simulink model "New_com_Fixed_Angle"  (R2025a)
settings: Solver=VariableStepAuto  StartTime=0.0  StopTime=Inf  RelTol=1e-3
values from neighbouring files (symbols this model uses):
  Boom_Cmd_LUT = joints(1).lut_y    [LUT.m]
  Boom_Vel_LUT = joints(1).lut_x    [LUT.m]
  Stick_Cmd_LUT = joints(2).lut_y    [LUT.m]
  Stick_Vel_LUT = joints(2).lut_x    [LUT.m]
undefined symbols (not defined in the file or in its folder): canChannel
libraries: canlib x10, canmsglib x8, simulink_extras x6, simulink x6, eeGeneralControl x5, slpidlib x5, aerolibanimutils x1, sl3dlib x1
(part 1 of 2)
settings Model: Creator=Viktor Traktor  LastModifiedBy=Viktor Traktor

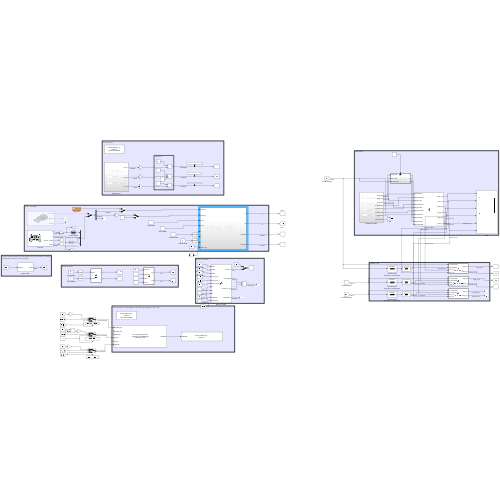
[thumbnail: Simulink's stored preview of the top-level diagram]
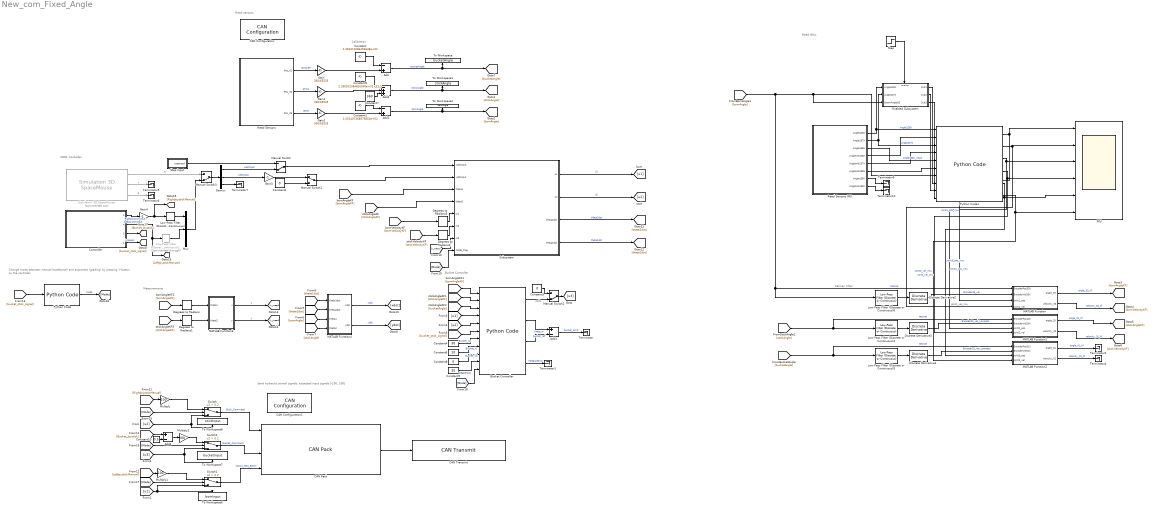
== system New_com_Fixed_Angle ==
  note: Change mode between manual (traditional) and automatic (grading)
      | by pressing Y-button on the controller
  note: Measurements
  note: Bucket Controller
  note: 2DOF Controller
  note: Calibration
  note: Send hydraulic control signals, expected input signals [-100, 100]
  note: Read sensors
  note: Kalman Filter
  note: Read IMUs
  Add : Sum  Inputs=-+
  Add1 : Sum  Inputs=+-
  Add2 : Sum  Inputs=-+
  Add3 : Sum  Inputs=-++
  Add4 : Sum  Inputs=+-
  Bucket Controller : PythonCode  OutputCode=|  SampleTime=0.01
      | import numpy as np
      | from numpy import sign, abs
      | 
      | #### TUNING PARAMETERS
      | degpersec 
      | Ts = 0.01
      | 
      | BUCKET_STICK1 = 16
      | BUCKET_STICK2 = 32
      | if flag is None:
      |     flag = 1
      | 
      | ## Bucket Control Parameters
      | Kp_bucket = Kp
      | Ki_bucket = Ki
      | Kd_bucket = Kd
      | 
      | ## Bucket controller
      | calc_thetaw = theta1 + theta2 + theta3
      | 
      | 
      | if theta_ref is None:
      |     theta_ref = -20
      | 
      | if comp_flag_1 is None:
      |     comp_flag_1 = 0
      | 
      |     
      | 
      | 
      | if bucket_stick_signal == 0 and flag == 0:
      |     if comp_flag_1 == 1:
      |         theta_ref = calc_thetaw - 0.6
      |     else:
      |         theta_ref = calc_thetaw + 0.6
      |     bucket_error_integral_prev = 0
      |     bucket_error_integral = 0
      |     bucket_error_prev = 0
      |     flag = 1
      |     
      | 
      | if bucket_stick_signal == BUCKET_STICK1 or bucket_stick_signal == BUCKET_STICK2:
      |     if bucket_stick_signal == BUCKET_STICK1 + BUCKET_STICK2:
      |         pass
      |     else:
      | 
      |         flag = 0
      | 
      |         if bucket_stick_signal == BUCKET_STICK1:
      |             theta_ref -= degpersec * Ts 
      |             comp_flag_1 = 1
      | 
      |         elif bucket_stick_signal == BUCKET_STICK2:
      |             theta_ref += degpersec * Ts 
      |             comp_flag_1 = 0
      |     
      | bucket_error = theta_ref - calc_thetaw
      | 
      | if bucket_error_prev is None:
      |     bucket_error_prev = bucket_error
      | if bucket_error_integral_prev is None:
      |     bucket_error_integral_prev  = 0
      | 
      | # calculate integral
      | if mode_flag == 1:
      |     
      |     bucket_error_integral = 0
      |     bucket_error_integral_prev = 0
      | 
      | else:
      |     bucket_error_integral = (bucket_error + bucket_error_prev) * Ts / 2 + bucket_error_integral_prev
      | 
      |     bucket_error_integral_prev = bucket_error_integral
      | 
      | 
      | # calculate derivative
      | bucket_error_derivative = (bucket_error - bucket_error_prev) / Ts
      | bucket_error_prev = bucket_error
      | 
      | 
      | control_3 = -(Kp_bucket * bucket_error +  Ki_bucket * bucket_error_integral +  Kd_bucket * bucket_error_derivative  + 0.2*stick_input + 0.2*bom_input)
      | control_3 = np.clip(control_3,-99, 90)
      | #if control_3 < 0:
      | #    control_3 = control_3 * 0.85 - 15
      | #else:
      | #    control_3 = control_3 * 0.85 + 15
      |             
      | bucket_ref_out = theta_ref
      | 
      | IntegralError = bucket_error_integral
  CAN Configuration : canlib/CAN Configuration  BlockHandle=316.0001  Device=Kvaser USBcan Light 1 (Channel 1)  DeviceMenu=Kvaser USBcan Light 1 (Channel 1)  ObjConstructor=canChannel('Kvaser', 'USBcan Light 1', 1)  BusSpeed=500000  EnableBitParameters=off  SJW=1  TSEG1=4  TSEG2=3  NSamples=1  AckMode=Normal
  CAN Configuration1 : canlib/CAN Configuration  BlockHandle=317.0001  Device=Kvaser USBcan Light 1 (Channel 2)  DeviceMenu=Kvaser USBcan Light 1 (Channel 2)  ObjConstructor=canChannel('Kvaser', 'USBcan Light 1', 2)  BusSpeed=500000  EnableBitParameters=off  SJW=1  TSEG1=4  TSEG2=3  NSamples=1  AckMode=Normal
  CAN Pack : canmsglib/CAN Pack  CANdbFile=C:\Users\Viktor Traktor\IQAN\ec20_hydraulics.dbc  MsgList=ControlMessage  MsgName=ControlMessage  MsgIDType=Standard (11-bit identifier)  MsgIdentifier=387  CANIDInput=off  MsgLength=6  Remote=off  ApplyMinMax=off  BusOutput=off  SignalInfo={'Parallell_FR','8','8','LE','signed','Standard','0','1','0','-Inf','Inf';'Parallelll_RL','0','8','LE','signed','Standard','0','1','0','-Inf','Inf';'Rotate_RL','40','8','LE','signed','Standard','0','1','0','-Inf','Inf';'Tilt_FR','24','8','LE','signed','Standard','0','1','0','-Inf','Inf';'Tilt_RL','32','8','LE','signed','Standard','0','1','0','-Inf','Inf';'UpDown','16','8','LE','signed','Standard','0','1','0','-Inf','Inf'}
      settings: LibrarySourceBlock=canlib/CAN Pack  DataFormat=CANdb specified signals
  CAN Transmit : canlib/CAN Transmit  BlockHandle=326.0001  Device=Kvaser USBcan Light 1 (Channel 2)  DeviceMenu=Kvaser USBcan Light 1 (Channel 2)  ObjConstructor=canChannel('Kvaser', 'USBcan Light 1', 2)  EnableEventTransmit=off  EnablePeriodicTransmit=off  MessagePeriod=1.000
  Constant : Constant  Value=2.060410383456638e+02
  Constant1 : Constant  Value=2.052407368979854e+02
  Constant10 : Constant  Value=0.5
  Constant2 : Constant  Value=0
  Constant3 : Constant  Value=0
  Constant4 : Constant  Value=30
  Constant5 : Constant  Value=2.390501084826040e+02+27.5
  Constant6 : Constant  Value=10
  Constant7 : Constant  Value=360
  Constant8 : Constant  Value=0
  Constant9 : Constant  Value=30
  Controller : Subsystem
      mask Display: image('controller.png', [0,0,20,0,100,100]);
  Degrees to Radians{,1..2,5} (4 alike) : simulink_extras/Transformations/Degrees to Radians
  Demux : Demux  Outputs=3
  Discrete Derivative2 : simulink/Discrete/Discrete Derivative  gainval=1.0  ICPrevScaledInput=0.0  OutMin=[]  OutMax=[]  OutDataType=fixdt(1, 16)  OutScaling=2^-10  DoSatur=off
  Discrete Derivative3 : simulink/Discrete/Discrete Derivative  gainval=1.0  ICPrevScaledInput=0.0  OutMin=[]  OutMax=[]  OutDataType=fixdt(1, 16)  OutScaling=2^-10  DoSatur=off
  Discrete Derivative4 : simulink/Discrete/Discrete Derivative  gainval=1.0  ICPrevScaledInput=0.0  OutMin=[]  OutMax=[]  OutDataType=fixdt(1, 16)  OutScaling=2^-10  DoSatur=off
  Enabled Subsystem : Subsystem  TreatAsAtomicUnit=on
  Gain : Gain  Gain=360/65535
  Gain1 : Gain  Gain=360/65535
  Gain2 : Gain  Gain=360/65535
  Gain3 : Gain  Gain=-1
  Gain4 : Gain  Gain=-1
  IMU : Scope  NumInputPorts=6
      settings: ActiveDisplayYMinimum=240.03476604985391  ActiveDisplayYMaximum=241.62685406904103
  Low-Pass Filter (Discrete or Continuous) : eeGeneralControl/Low-Pass Filter (Discrete or Continuous)  K=1  T=0.2  B=inf  A=-inf  init_option=Inherited from block input  x0=0  Ts=-1
  Low-Pass Filter (Discrete or Continuous)1 : eeGeneralControl/Low-Pass Filter (Discrete or Continuous)  Commented=through  K=1  T=0.2  B=inf  A=-inf  init_option=Inherited from block input  x0=0  Ts=-1
  Low-Pass Filter (Discrete or Continuous)4 : eeGeneralControl/Low-Pass Filter (Discrete or Continuous)  K=1  T=.15  B=inf  A=-inf  init_option=Inherited from block input  x0=0  Ts=0.1
  Low-Pass Filter (Discrete or Continuous)5 : eeGeneralControl/Low-Pass Filter (Discrete or Continuous)  K=1  T=.15  B=inf  A=-inf  init_option=Inherited from block input  x0=0  Ts=0.1
  Low-Pass Filter (Discrete or Continuous)6 : eeGeneralControl/Low-Pass Filter (Discrete or Continuous)  K=1  T=.15  B=inf  A=-inf  init_option=Inherited from block input  x0=0  Ts=0.1
  MATLAB Function : MATLAB Function  TreatAsAtomicUnit=on
  MATLAB Function1 : MATLAB Function  TreatAsAtomicUnit=on
  MATLAB Function2 : MATLAB Function  TreatAsAtomicUnit=on
  MATLAB Function3 : MATLAB Function  TreatAsAtomicUnit=on
  MATLAB Function4 : MATLAB Function  TreatAsAtomicUnit=on
  Manual Switch : ManualSwitch  CurrentSetting=0
  Manual Switch1 : ManualSwitch
  Manual Switch2 : ManualSwitch  CurrentSetting=0
  Manual Switch3 : ManualSwitch  CurrentSetting=0
  Multiply : Gain  Gain=100
  Multiply1 : Gain  Gain=100
  Multiply2 : Gain  Gain=200
  Mux : Mux  Inputs=3
  Python Code : PythonCode  OutputCode=|
      | if flag is None:
      |     flag = 1
      |     mode = 0
      | 
      | # Detect button press
      | if knapp_Y == 8 and flag == 1:
      |     mode = 1 if mode == 0 else 0  # toggle mode
      |     flag = 0                       # mark the press as handled
      | 
      | 
      | # Reset the flag when button is released
      | if knapp_Y != 8:
      |     flag = 1
  Python Code1 : PythonCode  OutputCode=|  SampleTime=0.01
      | # Computation
      | 
      | #print(Angle128X)
      | 
      | if Angle128X > 180:
      |     Angle128X = abs(Angle128X) - 360
      |     
      | if Angle137X < 20:
      |     Angle137X = abs(Angle137X)+360
      |     
      | if Angle138X > 270:
      |     Angle138X = abs(Angle138X) - 360
      |     
      | #print("///")
      | #print(Angle128X)
      | 
      | print(Angle128Xp)
      | print(Angle137Xp)
      | print(Encoder33Xp)
      |     
      | joint1_pos = Angle137X -270 + Angle128X - (Angle137Xp-270 + Angle128Xp - Encoder33Xp)
      | joint1_vel = -(AngleVel137X - AngleVel128X)
      | 
      | joint2_pos = 180 + (90 - joint1_pos) + Angle138X
      | joint2_vel = AngleVel138X - joint1_vel
      | 
      | joint3_pos = 0
      | joint3_vel = 0
  Read Sensors : Subsystem
  Read Sensors IMU : Subsystem
  Simulation 3D SpaceMouse : sl3dlib/Simulation 3D/Hardware Interface/Simulation 3D SpaceMouse  Commented=on  Port=USB1  OutputType=Speed  Dominant=off  DisableTranslation=off  DisableRotation=off  NormalizeAngle=off  EnableLimit=off  PositionSensitivity=0.00058  RotationSensitivity=0.00001  InitialPosition=[0 0 0]  InitialRotation=[0 0 1 0]  PositionLow=[-100 -100 -100]  PositionUp=[100 100 100]
  Step : Step  Time=0.001  Before=1  After=0  SampleTime=0
  Step Input : Subsystem
  Subsystem : Subsystem
  Switch : Switch  Criteria=u2 > Threshold  Threshold=0.2  SaturateOnIntegerOverflow=off  InputSameDT=off
  Switch1 : Switch  Criteria=u2 > Threshold  Threshold=0.2  SaturateOnIntegerOverflow=off  InputSameDT=off
  Switch2 : Switch  Criteria=u2 > Threshold  Threshold=0.2  SaturateOnIntegerOverflow=off  InputSameDT=off
  Terminator{,1..2,4..7,9..10} (9 alike) : Terminator
  To Workspace : ToWorkspace  VariableName=bucketAngle  SaveFormat=Timeseries  SampleTime=-1
  To Workspace1 : ToWorkspace  VariableName=stickAngle  SaveFormat=Timeseries  SampleTime=-1
  To Workspace2 : ToWorkspace  VariableName=bomAngle  SaveFormat=Timeseries  SampleTime=-1
  To Workspace6 : ToWorkspace  VariableName=bomInput  SaveFormat=Timeseries  SampleTime=-1
  To Workspace7 : ToWorkspace  VariableName=bucketInput  SaveFormat=Timeseries  SampleTime=-1
  To Workspace8 : ToWorkspace  VariableName=stickInput  SaveFormat=Timeseries  SampleTime=-1
  wires:
  [u3] -> Switch2/3, To Workspace7/1
  Add2/1 -> [bomAngle], To Workspace2/1  "bomAngle"
  Constant1/1 -> Add2/1
  Gain/1 -> Add/2
  Read Sensors/2(Pos_20) -> Gain1/1  "STICK"
  [u2] -> To Workspace8/1, Switch/3
  Constant/1 -> Add/1
  Read Sensors/1(Pos_01) -> Gain/1  "BUCKET"
  Gain2/1 -> Add2/2
  Read Sensors/3(Pos_33) -> Gain2/1  "BOM"
  CAN Pack/1 -> CAN Transmit/1
  Add/1 -> [bucketAngle], To Workspace/1  "bucketAngle"
  [u1] -> To Workspace6/1, Switch1/3
  Add3/1 -> [stickAngle], To Workspace1/1  "stickAngle"
  MATLAB Function1/2(velocity_20) -> [stickVelocityKF]  "velocity_20_kf"
  Enabled Subsystem/1(Out1) -> Python Code1/8
  Discrete Derivative2/1 -> MATLAB Function/2(EncoderVel33X)  "Encoder33_vel"
  MATLAB Function/1(angle_33) -> [bomAngleKF]  "angle_33_kf"
  Read Sensors IMU/3(Angle138X) -> Python Code1/5  "Angle138X_input"
  Python Code1/4 -> MATLAB Function1/4(joint2_vel), IMU/4  "join2_vel_imu"
  Read Sensors IMU/4(AngleVel128X) -> Python Code1/2
  Read Sensors IMU/1(Angle128X) -> Python Code1/1, Enabled Subsystem/1(Angle128X)  "Angle128X"
  Read Sensors IMU/8(AngleVel139X) -> Terminator10/1
  Python Code1/3 -> MATLAB Function1/3(joint2_pos), IMU/3  "joint2_pos_imu"
  Python Code1/5 -> MATLAB Function2/3(joint3_pos), IMU/5  "joint3_pos_imu"
  MATLAB Function/2(velocity_33) -> [bomVelocityKF]  "velocity_33_kf"
  Python Code1/6 -> MATLAB Function2/4(joint3_vel), IMU/6  "joint3_vel_imu"
  Python Code1/2 -> MATLAB Function/4(joint1_vel), IMU/2  "joint1_vel_imu"
  MATLAB Function1/1(angle_20) -> [stickAngleKF]  "anlge_20_kf"
  Enabled Subsystem/3(Out3) -> Python Code1/10
  Read Sensors IMU/2(Angle137X) -> Python Code1/3, Enabled Subsystem/2(Angle137X)  "Angle137X"
  Step/1 -> Enabled Subsystem/Enable
  Discrete Derivative3/1 -> MATLAB Function1/2(EncoderVel20X)  "Encoder20_vel_Lowpass"
  Read Sensors IMU/5(AngleVel137X) -> Python Code1/4
  Python Code1/1 -> MATLAB Function/3(joint1_pos), IMU/1  "joint1_pos_imu"
  MATLAB Function2/1(angle_01) -> Terminator2/1  "angle_01_kf"
  Read Sensors IMU/7(Angle139X) -> Terminator9/1
  MATLAB Function2/2(velocity_01) -> Terminator4/1  "velocity_01_kf"
  Read Sensors IMU/6(AngleVel138X) -> Python Code1/6
  Enabled Subsystem/2(Out2) -> Python Code1/9
  Discrete Derivative4/1 -> MATLAB Function2/2(EncoderVel01X)  "Encoder01_vel_Lowpass"
  Constant5/1 -> Add3/1
  Gain1/1 -> Add3/2
  Constant7/1 -> Add3/3
  [stickAngle] -> MATLAB Function1/1(EncoderPos20X), Low-Pass Filter (Discrete or Continuous)4/1  "testvel"
  [bomAngle] -> Low-Pass Filter (Discrete or Continuous)6/1, MATLAB Function/1(EncoderPos33X), Python Code1/7, Enabled Subsystem/3(BoomAngle33)  "testvel"
  [bucketAngle] -> MATLAB Function2/1(EncoderPos01X), Low-Pass Filter (Discrete or Continuous)5/1  "testvel"
  Low-Pass Filter (Discrete or Continuous)5/1 -> Discrete Derivative4/1
  Low-Pass Filter (Discrete or Continuous)4/1 -> Discrete Derivative3/1
  Low-Pass Filter (Discrete or Continuous)6/1 -> Discrete Derivative2/1
  Simulation 3D SpaceMouse/1 -> Manual Switch3/1  "tr"
  Subsystem/2(u2) -> [u2]  "u2"
  Demux/2 -> Gain3/1  "ydotInput"
  Demux/1 -> Manual Switch/2  "xdotInput"
  Simulation 3D SpaceMouse/2 -> Terminator5/1  "r"
  Simulation 3D SpaceMouse/3 -> Terminator6/1  "b"
  Subsystem/1(u1) -> [u1]  "u1"
  Gain3/1 -> Manual Switch1/1
  [bomAngleKF] -> Subsystem/3(theta1)
  [stickAngleKF] -> Subsystem/4(theta2)
  Degrees to Radians2/1 -> Subsystem/6(In2)
  [stickVelocityKF] -> Degrees to Radians2/1
  [bomVelocityKF] -> Degrees to Radians5/1
  Degrees to Radians5/1 -> Subsystem/5(In1)
  Step Input/1(stepInput) -> Manual Switch/1
  Manual Switch/1 -> Subsystem/1(xdotInput)
  Constant2/1 -> Manual Switch1/2
  Manual Switch1/1 -> Subsystem/2(ydotInput)
  Controller/2(4) -> Low-Pass Filter (Discrete or Continuous)1/1, [LeftJoystickManual]  "LeftJoystckInput"
  Controller/1(2) -> Gain4/1  "RightJoystickInput"
  Gain4/1 -> [RightJoystickManual], Low-Pass Filter (Discrete or Continuous)/1
  Mux/1 -> Manual Switch3/2
  Manual Switch3/1 -> Demux/1
  Controller/4(1) -> [bucket_stick_signal]  "knappar"
  Demux/3 -> Terminator7/1
  Subsystem/3(theta2dot) -> [theta2dot]  "theta2dot"
  Subsystem/4(theta1dot) -> [theta1dot]  "theta1dot"
  [y_meas] -> Subsystem/7(In3)
  Constant3/1 -> Manual Switch2/1
  [stickAngleKF] -> Bucket Controller/2
  [bomAngleKF] -> Bucket Controller/1
  [bucketAngle] -> Bucket Controller/3
  [u2] -> Bucket Controller/5
  [u1] -> Bucket Controller/4
  Bucket Controller/2 -> Add1/1  "theta_w"
  Manual Switch2/1 -> [u3]
  [bucket_stick_signal] -> Bucket Controller/6
  Bucket Controller/1 -> Manual Switch2/2  "ctrl3"
  Degrees to Radians1/1 -> MATLAB Function3/2(theta2)
  [bomAngleKF] -> Degrees to Radians/1
  [bomAngle] -> MATLAB Function4/3(theta1)
  [theta2dot] -> MATLAB Function4/2(theta2dot)
  [stickAngleKF] -> Degrees to Radians1/1
  MATLAB Function3/1(x) -> [x_meas]  "x"
  MATLAB Function4/2(ydot) -> [ydot]  "ydot"
  [theta1dot] -> MATLAB Function4/1(theta1dot)
  MATLAB Function3/2(y) -> [y_meas]  "y"
  [stickAngle] -> MATLAB Function4/4(theta2)
  MATLAB Function4/1(xdot) -> [xdot]  "xdot"
  Degrees to Radians/1 -> MATLAB Function3/1(theta1)
  Constant4/1 -> Bucket Controller/7  "Bucket_kp"
  Constant6/1 -> Bucket Controller/8  "Bucket_ki"
  Constant8/1 -> Bucket Controller/9  "Bucket_kd"
  Bucket Controller/3 -> Add1/2  "bucket_ref"
  Constant9/1 -> Bucket Controller/10  "Degpersec"
  Low-Pass Filter (Discrete or Continuous)1/1 -> Mux/2
  Low-Pass Filter (Discrete or Continuous)/1 -> Mux/1
  Add1/1 -> Terminator/1  "bucket_error"
  Switch/1 -> CAN Pack/1  "Stick_Command"
  Multiply/1 -> Switch/1
  [LeftJoystickManual] -> Multiply1/1
  Switch1/1 -> CAN Pack/6  "Marko_test_Boom"
  Multiply1/1 -> Switch1/1
  [bucket_stick_signal] -> Python Code/1
  [RightJoystickManual] -> Multiply/1
  Controller/3(3) -> [Bucket_Joystick]
  Python Code/1 -> [Mode]  "Mode"
  [Mode] -> Switch/2
  Multiply2/1 -> Switch2/1
  [Mode] -> Switch2/2
  [Mode] -> Switch1/2
  Switch2/1 -> CAN Pack/4  "Bucket_Command"
  Add4/1 -> Multiply2/1
  [Bucket_Joystick] -> Add4/1
  Constant10/1 -> Add4/2
  [Mode] -> Bucket Controller/11
  Bucket Controller/4 -> Terminator1/1  "IntegralError"
  [Mode] -> Subsystem/8(Mode_Flag)

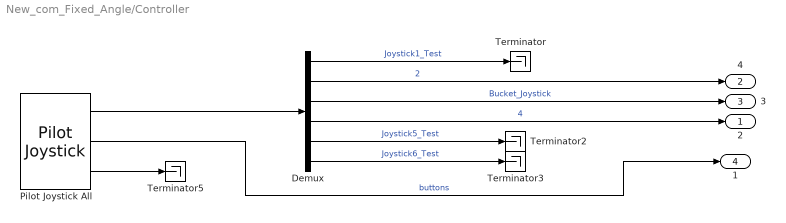
== system New_com_Fixed_Angle/Controller ==
  Demux : Demux  Outputs=6
  Pilot Joystick All : aerolibanimutils/Pilot Joystick  JoystickID=Joystick2  OutputConfiguration=AllOutputs  SampleTime=1/50
      settings: LibrarySourceBlock=aerolibanimutils/Pilot Joystick All
  Terminator{,2..3,5} (4 alike) : Terminator
  2 : Outport
  4 : Outport  Port=2
  3 : Outport  Port=3
  1 : Outport  Port=4
  wires:
  Demux/6 -> Terminator3/1  "Joystick6_Test"
  Demux/5 -> Terminator2/1  "Joystick5_Test"
  Pilot Joystick All/3 -> Terminator5/1
  Pilot Joystick All/1 -> Demux/1
  Demux/1 -> Terminator/1  "Joystick1_Test"
  Demux/4 -> 2/1  "4"
  Pilot Joystick All/2 -> 1/1  "buttons"
  Demux/3 -> 3/1  "Bucket_Joystick"
  Demux/2 -> 4/1  "2"

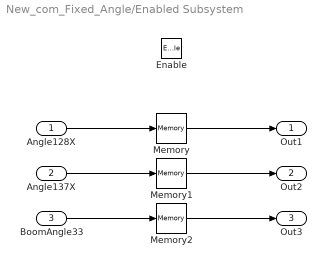
== system New_com_Fixed_Angle/Enabled Subsystem ==
  Angle128X : Inport
  Angle137X : Inport  Port=2
  BoomAngle33 : Inport  Port=3
  Enable : EnablePort
  Memory : Memory
  Memory1 : Memory
  Memory2 : Memory
  Out1 : Outport
  Out2 : Outport  Port=2
  Out3 : Outport  Port=3
  wires:
  Angle128X/1 -> Memory/1
  Memory/1 -> Out1/1
  Angle137X/1 -> Memory1/1
  BoomAngle33/1 -> Memory2/1
  Memory1/1 -> Out2/1
  Memory2/1 -> Out3/1

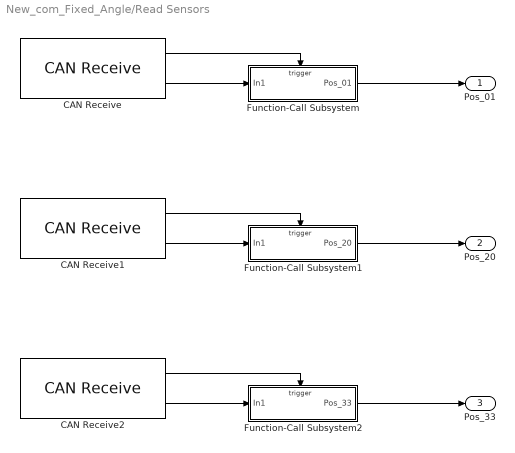
== system New_com_Fixed_Angle/Read Sensors ==
  CAN Receive : canlib/CAN Receive  BlockHandle=820.0001  Device=Kvaser USBcan Light 1 (Channel 1)  DeviceMenu=Kvaser USBcan Light 1 (Channel 1)  ObjConstructor=canChannel('Kvaser', 'USBcan Light 1', 1)  EnableStandardIDsFilter=off  StdIDsCombo=Allow all  StandardIDs=0  EnableExtendedIDsFilter=off  ExtIDsCombo=Allow all  ExtendedIDs=0  SampleTime=0.01  MsgsPerTimestep=all  InternalFilterUpdateStatus=on  BusOutput=off
  CAN Receive1 : canlib/CAN Receive  BlockHandle=823.0001  Device=Kvaser USBcan Light 1 (Channel 1)  DeviceMenu=Kvaser USBcan Light 1 (Channel 1)  ObjConstructor=canChannel('Kvaser', 'USBcan Light 1', 1)  EnableStandardIDsFilter=off  StdIDsCombo=Allow all  StandardIDs=0  EnableExtendedIDsFilter=off  ExtIDsCombo=Allow all  ExtendedIDs=0  SampleTime=0.01  MsgsPerTimestep=all  InternalFilterUpdateStatus=on  BusOutput=off
  CAN Receive2 : canlib/CAN Receive  BlockHandle=826.0001  Device=Kvaser USBcan Light 1 (Channel 1)  DeviceMenu=Kvaser USBcan Light 1 (Channel 1)  ObjConstructor=canChannel('Kvaser', 'USBcan Light 1', 1)  EnableStandardIDsFilter=off  StdIDsCombo=Allow all  StandardIDs=0  EnableExtendedIDsFilter=off  ExtIDsCombo=Allow all  ExtendedIDs=0  SampleTime=0.01  MsgsPerTimestep=all  InternalFilterUpdateStatus=on  BusOutput=off
  Function-Call Subsystem : Subsystem  TreatAsAtomicUnit=on
  Function-Call Subsystem1 : Subsystem  TreatAsAtomicUnit=on
  Function-Call Subsystem2 : Subsystem  TreatAsAtomicUnit=on
  Pos_01 : Outport
  Pos_20 : Outport  Port=2
  Pos_33 : Outport  Port=3
  wires:
  CAN Receive/2 -> Function-Call Subsystem/1(In1)
  CAN Receive1/2 -> Function-Call Subsystem1/1(In1)
  CAN Receive/1 -> Function-Call Subsystem/Trigger
  CAN Receive2/2 -> Function-Call Subsystem2/1(In1)
  Function-Call Subsystem2/1(Pos_33) -> Pos_33/1
  Function-Call Subsystem/1(Pos_01) -> Pos_01/1
  CAN Receive2/1 -> Function-Call Subsystem2/Trigger
  CAN Receive1/1 -> Function-Call Subsystem1/Trigger
  Function-Call Subsystem1/1(Pos_20) -> Pos_20/1

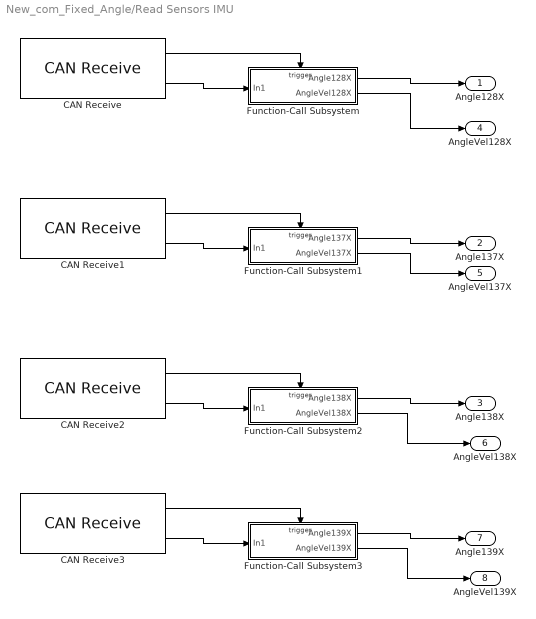
== system New_com_Fixed_Angle/Read Sensors IMU ==
  CAN Receive : canlib/CAN Receive  BlockHandle=907.0001  Device=Kvaser USBcan Light 1 (Channel 1)  DeviceMenu=Kvaser USBcan Light 1 (Channel 1)  ObjConstructor=canChannel('Kvaser', 'USBcan Light 1', 1)  EnableStandardIDsFilter=off  StdIDsCombo=Allow all  StandardIDs=0  EnableExtendedIDsFilter=off  ExtIDsCombo=Allow all  ExtendedIDs=0  SampleTime=0.01  MsgsPerTimestep=all  InternalFilterUpdateStatus=on  BusOutput=off
  CAN Receive1 : canlib/CAN Receive  BlockHandle=910.0001  Device=Kvaser USBcan Light 1 (Channel 1)  DeviceMenu=Kvaser USBcan Light 1 (Channel 1)  ObjConstructor=canChannel('Kvaser', 'USBcan Light 1', 1)  EnableStandardIDsFilter=off  StdIDsCombo=Allow all  StandardIDs=0  EnableExtendedIDsFilter=off  ExtIDsCombo=Allow all  ExtendedIDs=0  SampleTime=0.01  MsgsPerTimestep=all  InternalFilterUpdateStatus=on  BusOutput=off
  CAN Receive2 : canlib/CAN Receive  BlockHandle=913.0001  Device=Kvaser USBcan Light 1 (Channel 1)  DeviceMenu=Kvaser USBcan Light 1 (Channel 1)  ObjConstructor=canChannel('Kvaser', 'USBcan Light 1', 1)  EnableStandardIDsFilter=off  StdIDsCombo=Allow all  StandardIDs=0  EnableExtendedIDsFilter=off  ExtIDsCombo=Allow all  ExtendedIDs=0  SampleTime=0.01  MsgsPerTimestep=all  InternalFilterUpdateStatus=on  BusOutput=off
  CAN Receive3 : canlib/CAN Receive  BlockHandle=916.0001  Device=Kvaser USBcan Light 1 (Channel 1)  DeviceMenu=Kvaser USBcan Light 1 (Channel 1)  ObjConstructor=canChannel('Kvaser', 'USBcan Light 1', 1)  EnableStandardIDsFilter=off  StdIDsCombo=Allow all  StandardIDs=0  EnableExtendedIDsFilter=off  ExtIDsCombo=Allow all  ExtendedIDs=0  SampleTime=0.01  MsgsPerTimestep=all  InternalFilterUpdateStatus=on  BusOutput=off
  Function-Call Subsystem : Subsystem  TreatAsAtomicUnit=on
  Function-Call Subsystem1 : Subsystem  TreatAsAtomicUnit=on
  Function-Call Subsystem2 : Subsystem  TreatAsAtomicUnit=on
  Function-Call Subsystem3 : Subsystem  TreatAsAtomicUnit=on
  Angle128X : Outport
  Angle137X : Outport  Port=2
  Angle138X : Outport  Port=3
  AngleVel128X : Outport  Port=4
  AngleVel137X : Outport  Port=5
  AngleVel138X : Outport  Port=6
  Angle139X : Outport  Port=7
  AngleVel139X : Outport  Port=8
  wires:
  Function-Call Subsystem1/1(Angle137X) -> Angle137X/1
  CAN Receive1/1 -> Function-Call Subsystem1/Trigger
  CAN Receive2/1 -> Function-Call Subsystem2/Trigger
  Function-Call Subsystem/1(Angle128X) -> Angle128X/1
  Function-Call Subsystem2/1(Angle138X) -> Angle138X/1
  CAN Receive2/2 -> Function-Call Subsystem2/1(In1)
  CAN Receive/1 -> Function-Call Subsystem/Trigger
  CAN Receive1/2 -> Function-Call Subsystem1/1(In1)
  CAN Receive/2 -> Function-Call Subsystem/1(In1)
  Function-Call Subsystem/2(AngleVel128X) -> AngleVel128X/1
  Function-Call Subsystem1/2(AngleVel137X) -> AngleVel137X/1
  Function-Call Subsystem2/2(AngleVel138X) -> AngleVel138X/1
  Function-Call Subsystem3/2(AngleVel139X) -> AngleVel139X/1
  CAN Receive3/2 -> Function-Call Subsystem3/1(In1)
  Function-Call Subsystem3/1(Angle139X) -> Angle139X/1
  CAN Receive3/1 -> Function-Call Subsystem3/Trigger

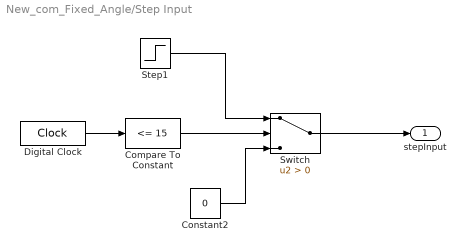
== system New_com_Fixed_Angle/Step Input ==
  Compare To Constant : simulink/Logic and Bit Operations/Compare To Constant  relop=<=  const=15  OutDataTypeStr=boolean
  Constant2 : Constant  Value=0
  Digital Clock : DigitalClock  SampleTime=0.01
  Step1 : Step  SampleTime=0.01
  Switch : Switch  Criteria=u2 > Threshold  SaturateOnIntegerOverflow=off  InputSameDT=off
  stepInput : Outport
  wires:
  Switch/1 -> stepInput/1
  Compare To Constant/1 -> Switch/2
  Digital Clock/1 -> Compare To Constant/1
  Step1/1 -> Switch/1
  Constant2/1 -> Switch/3

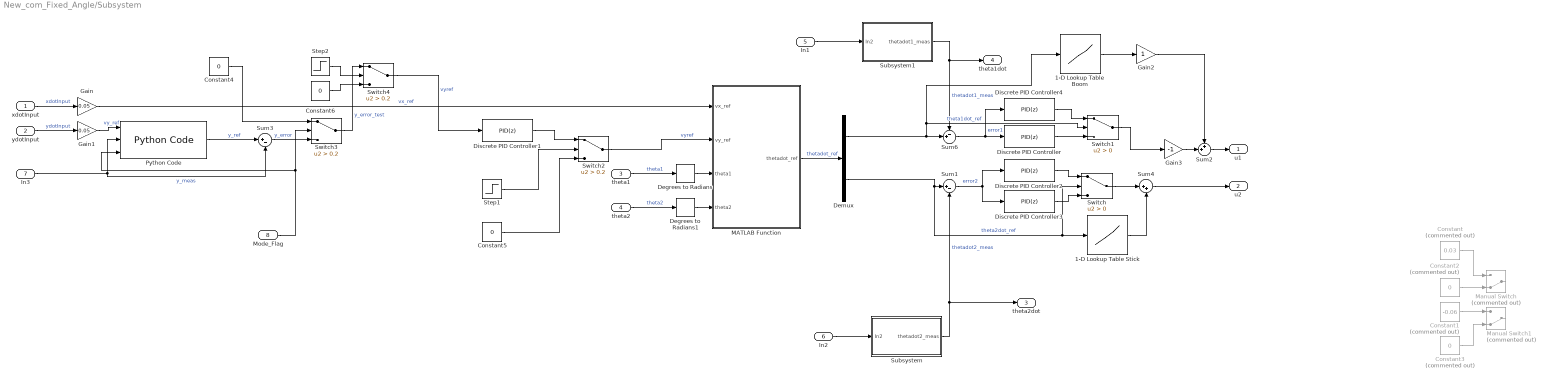
== system New_com_Fixed_Angle/Subsystem ==
  xdotInput : Inport
  ydotInput : Inport  Port=2
  theta1 : Inport  Port=3
  theta2 : Inport  Port=4
  In1 : Inport  Port=5
  In2 : Inport  Port=6
  In3 : Inport  Port=7
  Mode_Flag : Inport  Port=8
  1-D Lookup Table Boom : Lookup_n-D  NumberOfTableDimensions=1  BreakpointsForDimension1=Boom_Vel_LUT  Table=Boom_Cmd_LUT  InternalRulePriority=Speed  RndMeth=Simplest
  1-D Lookup Table Stick : Lookup_n-D  NumberOfTableDimensions=1  BreakpointsForDimension1=Stick_Vel_LUT  Table=Stick_Cmd_LUT  InternalRulePriority=Speed  RndMeth=Simplest
  Constant : Constant  Commented=on  Value=0.03
  Constant1 : Constant  Commented=on  Value=-0.06
  Constant2 : Constant  Commented=on  Value=0
  Constant3 : Constant  Commented=on  Value=0
  Constant4 : Constant  Value=0
  Constant5 : Constant  Value=0
  Constant6 : Constant  Value=0
  Degrees to Radians : simulink_extras/Transformations/Degrees to Radians
  Degrees to Radians1 : simulink_extras/Transformations/Degrees to Radians
  Demux : Demux  Outputs=2
  Discrete PID Controller : slpidlib/PID Controller  Controller=PID  Form=Parallel  TimeDomain=Discrete-time  UseExternalTs=off  SampleTime=-1  IntegratorMethod=Forward Euler  FilterMethod=Forward Euler  ControllerParametersSource=internal  P=75  I=100  UseKiTs=off  D=3  UseExternalDerivativeSource=off  N=100  UseFilter=on  TunerSelectOption=Transfer Function Based (PID Tuner App)  InitialConditionSource=internal  InitialConditionForIntegrator=0  InitialConditionForFilter=0  DifferentiatorICPrevScaledInput=0  ExternalReset=none  TrackingMode=off  Kt=1  LimitOutput=on  SatLimitsSource=internal  UpperSaturationLimit=100  LowerSaturationLimit=-100  LinearizeAsGain=off  AntiWindupMode=clamping  Kb=1  LimitIntegrator=on  UpperIntegratorSaturationLimit=50  LowerIntegratorSaturationLimit=-50  POutMin=[]  POutMax=[]  IOutMin=[]  IOutMax=[]  DOutMin=[]  DOutMax=[]  NOutMin=[]  NOutMax=[]  SumOutMin=[]  SumOutMax=[]  SaturationOutMin=[]  SaturationOutMax=[]  PParamMin=[]  PParamMax=[]  IParamMin=[]  IParamMax=[]  DParamMin=[]  DParamMax=[]  NParamMin=[]  NParamMax=[]  KbParamMin=[]  KbParamMax=[]  KtParamMin=[]  KtParamMax=[]  KbOutMin=[]  KbOutMax=[]  KtOutMin=[]  KtOutMax=[]  IntegratorOutMin=[]  IntegratorOutMax=[]  FilterOutMin=[]  FilterOutMax=[]  SumI1OutMin=[]  SumI1OutMax=[]  SumI2OutMin=[]  SumI2OutMax=[]  SumI3OutMin=[]  SumI3OutMax=[]  SumI4OutMin=[]  SumI4OutMax=[]  SumDOutMin=[]  SumDOutMax=[]  DifferentiatorOutMin=[]  DifferentiatorOutMax=[]  FilterDiffOutCoefMin=[]  FilterDiffOutCoefMax=[]  ReciprocalOutMin=[]  ReciprocalOutMax=[]  SumDenOutMin=[]  SumDenOutMax=[]  SumNumOutMin=[]  SumNumOutMax=[]  DivideOutMin=[]  DivideOutMax=[]  UdiffTsProdOutMin=[]  UdiffTsProdOutMax=[]  NTsProdOutMin=[]  NTsProdOutMax=[]  UintegralTsProdOutMin=[]  UintegralTsProdOutMax=[]  UngainTsProdOutMin=[]  UngainTsProdOutMax=[]  ClampingZeroOutDataTypeStr=Inherit: Inherit via back propagation  ClampingZeroOutMin=[]  ClampingZeroOutMax=[]  FilterDenConstantOutDataTypeStr=Inherit: Inherit via back propagation  FilterDenConstantOutMin=[]  FilterDenConstantOutMax=[]  PCopyOutDataTypeStr=Inherit: Inherit via back propagation  PCopyOutMin=[]  PCopyOutMax=[]  NCopyOutDataTypeStr=Inherit: Inherit via back propagation  NCopyOutMin=[]  NCopyOutMax=[]  IntegratorContinuousStateAttributes=''  IntegratorStateMustResolveToSignalObject=off  IntegratorRTWStateStorageClass=Auto  FilterContinuousStateAttributes=''  FilterStateMustResolveToSignalObject=off  FilterRTWStateStorageClass=Auto  ParallelPVariant=InternalParameters  IdealPVariant=Disabled  IVariant=InternalParameters  DVariant=InternalParameters  IntegratorVariant=Discrete  SatVariant=Enabled  AWVariant=DiscClampingParallel  PCopyVariant=Disabled  TRVariant=Disabled  FdbkBlocksVariant=Forward  IdealPFdbkVariant=Disabled  SatFdbkVariant=Disabled  DerivativeFilterVariant=ForwardEulerFilter  NVariant=InternalParameters  NCopyVariant=Disabled  FilterICVariant=InternalICsFilter  IntegratorICVariant=InternalICs  ExternalResetVariant=Disabled  TRSumVariant=Passthrough  SumFdbkVariant=Disabled  SumVariant=Sum_PID  TsampFilterVariant=InternalTs  TsampNgainVariant=Passthrough  TsampIntegralVariant=Disabled_SignalSpec  ExternalSaturationOutDataTypeStr=Inherit: Same as second input  DerivativeSourceVariant=ErrorSignal  PreIntVariant=InternalPreInt
      settings: LibrarySourceBlock=simulink/Discrete/Discrete PID Controller
  Discrete PID Controller1 : slpidlib/PID Controller  Controller=PID  Form=Parallel  TimeDomain=Discrete-time  UseExternalTs=off  SampleTime=-1  IntegratorMethod=Forward Euler  FilterMethod=Forward Euler  ControllerParametersSource=internal  P=1.3  I=0.8  UseKiTs=off  D=0  UseExternalDerivativeSource=off  N=30  UseFilter=on  TunerSelectOption=Transfer Function Based (PID Tuner App)  InitialConditionSource=internal  InitialConditionForIntegrator=0  InitialConditionForFilter=0  DifferentiatorICPrevScaledInput=0  ExternalReset=none  TrackingMode=off  Kt=1  LimitOutput=on  SatLimitsSource=internal  UpperSaturationLimit=100  LowerSaturationLimit=-100  LinearizeAsGain=off  AntiWindupMode=clamping  Kb=1  LimitIntegrator=on  UpperIntegratorSaturationLimit=50  LowerIntegratorSaturationLimit=-50  POutMin=[]  POutMax=[]  IOutMin=[]  IOutMax=[]  DOutMin=[]  DOutMax=[]  NOutMin=[]  NOutMax=[]  SumOutMin=[]  SumOutMax=[]  SaturationOutMin=[]  SaturationOutMax=[]  PParamMin=[]  PParamMax=[]  IParamMin=[]  IParamMax=[]  DParamMin=[]  DParamMax=[]  NParamMin=[]  NParamMax=[]  KbParamMin=[]  KbParamMax=[]  KtParamMin=[]  KtParamMax=[]  KbOutMin=[]  KbOutMax=[]  KtOutMin=[]  KtOutMax=[]  IntegratorOutMin=[]  IntegratorOutMax=[]  FilterOutMin=[]  FilterOutMax=[]  SumI1OutMin=[]  SumI1OutMax=[]  SumI2OutMin=[]  SumI2OutMax=[]  SumI3OutMin=[]  SumI3OutMax=[]  SumI4OutMin=[]  SumI4OutMax=[]  SumDOutMin=[]  SumDOutMax=[]  DifferentiatorOutMin=[]  DifferentiatorOutMax=[]  FilterDiffOutCoefMin=[]  FilterDiffOutCoefMax=[]  ReciprocalOutMin=[]  ReciprocalOutMax=[]  SumDenOutMin=[]  SumDenOutMax=[]  SumNumOutMin=[]  SumNumOutMax=[]  DivideOutMin=[]  DivideOutMax=[]  UdiffTsProdOutMin=[]  UdiffTsProdOutMax=[]  NTsProdOutMin=[]  NTsProdOutMax=[]  UintegralTsProdOutMin=[]  UintegralTsProdOutMax=[]  UngainTsProdOutMin=[]  UngainTsProdOutMax=[]  ClampingZeroOutDataTypeStr=Inherit: Inherit via back propagation  ClampingZeroOutMin=[]  ClampingZeroOutMax=[]  FilterDenConstantOutDataTypeStr=Inherit: Inherit via back propagation  FilterDenConstantOutMin=[]  FilterDenConstantOutMax=[]  PCopyOutDataTypeStr=Inherit: Inherit via back propagation  PCopyOutMin=[]  PCopyOutMax=[]  NCopyOutDataTypeStr=Inherit: Inherit via back propagation  NCopyOutMin=[]  NCopyOutMax=[]  IntegratorContinuousStateAttributes=''  IntegratorStateMustResolveToSignalObject=off  IntegratorRTWStateStorageClass=Auto  FilterContinuousStateAttributes=''  FilterStateMustResolveToSignalObject=off  FilterRTWStateStorageClass=Auto  ParallelPVariant=InternalParameters  IdealPVariant=Disabled  IVariant=InternalParameters  DVariant=InternalParameters  IntegratorVariant=Discrete  SatVariant=Enabled  AWVariant=DiscClampingParallel  PCopyVariant=Disabled  TRVariant=Disabled  FdbkBlocksVariant=Forward  IdealPFdbkVariant=Disabled  SatFdbkVariant=Disabled  DerivativeFilterVariant=ForwardEulerFilter  NVariant=InternalParameters  NCopyVariant=Disabled  FilterICVariant=InternalICsFilter  IntegratorICVariant=InternalICs  ExternalResetVariant=Disabled  TRSumVariant=Passthrough  SumFdbkVariant=Disabled  SumVariant=Sum_PID  TsampFilterVariant=InternalTs  TsampNgainVariant=Passthrough  TsampIntegralVariant=Disabled_SignalSpec  ExternalSaturationOutDataTypeStr=Inherit: Same as second input  DerivativeSourceVariant=ErrorSignal  PreIntVariant=InternalPreInt
      settings: LibrarySourceBlock=simulink/Discrete/Discrete PID Controller
  Discrete PID Controller2 : slpidlib/PID Controller  Controller=PID  Form=Parallel  TimeDomain=Discrete-time  UseExternalTs=off  SampleTime=-1  IntegratorMethod=Forward Euler  FilterMethod=Forward Euler  ControllerParametersSource=internal  P=80  I=85  UseKiTs=off  D=0  UseExternalDerivativeSource=off  N=100  UseFilter=on  TunerSelectOption=Transfer Function Based (PID Tuner App)  InitialConditionSource=internal  InitialConditionForIntegrator=0  InitialConditionForFilter=0  DifferentiatorICPrevScaledInput=0  ExternalReset=none  TrackingMode=off  Kt=1  LimitOutput=on  SatLimitsSource=internal  UpperSaturationLimit=100  LowerSaturationLimit=-100  LinearizeAsGain=off  AntiWindupMode=clamping  Kb=1  LimitIntegrator=on  UpperIntegratorSaturationLimit=50  LowerIntegratorSaturationLimit=-50  POutMin=[]  POutMax=[]  IOutMin=[]  IOutMax=[]  DOutMin=[]  DOutMax=[]  NOutMin=[]  NOutMax=[]  SumOutMin=[]  SumOutMax=[]  SaturationOutMin=[]  SaturationOutMax=[]  PParamMin=[]  PParamMax=[]  IParamMin=[]  IParamMax=[]  DParamMin=[]  DParamMax=[]  NParamMin=[]  NParamMax=[]  KbParamMin=[]  KbParamMax=[]  KtParamMin=[]  KtParamMax=[]  KbOutMin=[]  KbOutMax=[]  KtOutMin=[]  KtOutMax=[]  IntegratorOutMin=[]  IntegratorOutMax=[]  FilterOutMin=[]  FilterOutMax=[]  SumI1OutMin=[]  SumI1OutMax=[]  SumI2OutMin=[]  SumI2OutMax=[]  SumI3OutMin=[]  SumI3OutMax=[]  SumI4OutMin=[]  SumI4OutMax=[]  SumDOutMin=[]  SumDOutMax=[]  DifferentiatorOutMin=[]  DifferentiatorOutMax=[]  FilterDiffOutCoefMin=[]  FilterDiffOutCoefMax=[]  ReciprocalOutMin=[]  ReciprocalOutMax=[]  SumDenOutMin=[]  SumDenOutMax=[]  SumNumOutMin=[]  SumNumOutMax=[]  DivideOutMin=[]  DivideOutMax=[]  UdiffTsProdOutMin=[]  UdiffTsProdOutMax=[]  NTsProdOutMin=[]  NTsProdOutMax=[]  UintegralTsProdOutMin=[]  UintegralTsProdOutMax=[]  UngainTsProdOutMin=[]  UngainTsProdOutMax=[]  ClampingZeroOutDataTypeStr=Inherit: Inherit via back propagation  ClampingZeroOutMin=[]  ClampingZeroOutMax=[]  FilterDenConstantOutDataTypeStr=Inherit: Inherit via back propagation  FilterDenConstantOutMin=[]  FilterDenConstantOutMax=[]  PCopyOutDataTypeStr=Inherit: Inherit via back propagation  PCopyOutMin=[]  PCopyOutMax=[]  NCopyOutDataTypeStr=Inherit: Inherit via back propagation  NCopyOutMin=[]  NCopyOutMax=[]  IntegratorContinuousStateAttributes=''  IntegratorStateMustResolveToSignalObject=off  IntegratorRTWStateStorageClass=Auto  FilterContinuousStateAttributes=''  FilterStateMustResolveToSignalObject=off  FilterRTWStateStorageClass=Auto  ParallelPVariant=InternalParameters  IdealPVariant=Disabled  IVariant=InternalParameters  DVariant=InternalParameters  IntegratorVariant=Discrete  SatVariant=Enabled  AWVariant=DiscClampingParallel  PCopyVariant=Disabled  TRVariant=Disabled  FdbkBlocksVariant=Forward  IdealPFdbkVariant=Disabled  SatFdbkVariant=Disabled  DerivativeFilterVariant=ForwardEulerFilter  NVariant=InternalParameters  NCopyVariant=Disabled  FilterICVariant=InternalICsFilter  IntegratorICVariant=InternalICs  ExternalResetVariant=Disabled  TRSumVariant=Passthrough  SumFdbkVariant=Disabled  SumVariant=Sum_PID  TsampFilterVariant=InternalTs  TsampNgainVariant=Passthrough  TsampIntegralVariant=Disabled_SignalSpec  ExternalSaturationOutDataTypeStr=Inherit: Same as second input  DerivativeSourceVariant=ErrorSignal  PreIntVariant=InternalPreInt
      settings: LibrarySourceBlock=simulink/Discrete/Discrete PID Controller
  Discrete PID Controller3 : slpidlib/PID Controller  Controller=PID  Form=Parallel  TimeDomain=Discrete-time  UseExternalTs=off  SampleTime=-1  IntegratorMethod=Forward Euler  FilterMethod=Forward Euler  ControllerParametersSource=internal  P=90  I=40  UseKiTs=off  D=2  UseExternalDerivativeSource=off  N=100  UseFilter=on  TunerSelectOption=Transfer Function Based (PID Tuner App)  InitialConditionSource=internal  InitialConditionForIntegrator=0  InitialConditionForFilter=0  DifferentiatorICPrevScaledInput=0  ExternalReset=none  TrackingMode=off  Kt=1  LimitOutput=on  SatLimitsSource=internal  UpperSaturationLimit=100  LowerSaturationLimit=-100  LinearizeAsGain=off  AntiWindupMode=clamping  Kb=1  LimitIntegrator=on  UpperIntegratorSaturationLimit=50  LowerIntegratorSaturationLimit=-50  POutMin=[]  POutMax=[]  IOutMin=[]  IOutMax=[]  DOutMin=[]  DOutMax=[]  NOutMin=[]  NOutMax=[]  SumOutMin=[]  SumOutMax=[]  SaturationOutMin=[]  SaturationOutMax=[]  PParamMin=[]  PParamMax=[]  IParamMin=[]  IParamMax=[]  DParamMin=[]  DParamMax=[]  NParamMin=[]  NParamMax=[]  KbParamMin=[]  KbParamMax=[]  KtParamMin=[]  KtParamMax=[]  KbOutMin=[]  KbOutMax=[]  KtOutMin=[]  KtOutMax=[]  IntegratorOutMin=[]  IntegratorOutMax=[]  FilterOutMin=[]  FilterOutMax=[]  SumI1OutMin=[]  SumI1OutMax=[]  SumI2OutMin=[]  SumI2OutMax=[]  SumI3OutMin=[]  SumI3OutMax=[]  SumI4OutMin=[]  SumI4OutMax=[]  SumDOutMin=[]  SumDOutMax=[]  DifferentiatorOutMin=[]  DifferentiatorOutMax=[]  FilterDiffOutCoefMin=[]  FilterDiffOutCoefMax=[]  ReciprocalOutMin=[]  ReciprocalOutMax=[]  SumDenOutMin=[]  SumDenOutMax=[]  SumNumOutMin=[]  SumNumOutMax=[]  DivideOutMin=[]  DivideOutMax=[]  UdiffTsProdOutMin=[]  UdiffTsProdOutMax=[]  NTsProdOutMin=[]  NTsProdOutMax=[]  UintegralTsProdOutMin=[]  UintegralTsProdOutMax=[]  UngainTsProdOutMin=[]  UngainTsProdOutMax=[]  ClampingZeroOutDataTypeStr=Inherit: Inherit via back propagation  ClampingZeroOutMin=[]  ClampingZeroOutMax=[]  FilterDenConstantOutDataTypeStr=Inherit: Inherit via back propagation  FilterDenConstantOutMin=[]  FilterDenConstantOutMax=[]  PCopyOutDataTypeStr=Inherit: Inherit via back propagation  PCopyOutMin=[]  PCopyOutMax=[]  NCopyOutDataTypeStr=Inherit: Inherit via back propagation  NCopyOutMin=[]  NCopyOutMax=[]  IntegratorContinuousStateAttributes=''  IntegratorStateMustResolveToSignalObject=off  IntegratorRTWStateStorageClass=Auto  FilterContinuousStateAttributes=''  FilterStateMustResolveToSignalObject=off  FilterRTWStateStorageClass=Auto  ParallelPVariant=InternalParameters  IdealPVariant=Disabled  IVariant=InternalParameters  DVariant=InternalParameters  IntegratorVariant=Discrete  SatVariant=Enabled  AWVariant=DiscClampingParallel  PCopyVariant=Disabled  TRVariant=Disabled  FdbkBlocksVariant=Forward  IdealPFdbkVariant=Disabled  SatFdbkVariant=Disabled  DerivativeFilterVariant=ForwardEulerFilter  NVariant=InternalParameters  NCopyVariant=Disabled  FilterICVariant=InternalICsFilter  IntegratorICVariant=InternalICs  ExternalResetVariant=Disabled  TRSumVariant=Passthrough  SumFdbkVariant=Disabled  SumVariant=Sum_PID  TsampFilterVariant=InternalTs  TsampNgainVariant=Passthrough  TsampIntegralVariant=Disabled_SignalSpec  ExternalSaturationOutDataTypeStr=Inherit: Same as second input  DerivativeSourceVariant=ErrorSignal  PreIntVariant=InternalPreInt
      settings: LibrarySourceBlock=simulink/Discrete/Discrete PID Controller
  Discrete PID Controller4 : slpidlib/PID Controller  Controller=PID  Form=Parallel  TimeDomain=Discrete-time  UseExternalTs=off  SampleTime=-1  IntegratorMethod=Forward Euler  FilterMethod=Forward Euler  ControllerParametersSource=internal  P=140  I=40  UseKiTs=off  D=0  UseExternalDerivativeSource=off  N=100  UseFilter=on  TunerSelectOption=Transfer Function Based (PID Tuner App)  InitialConditionSource=internal  InitialConditionForIntegrator=0  InitialConditionForFilter=0  DifferentiatorICPrevScaledInput=0  ExternalReset=none  TrackingMode=off  Kt=1  LimitOutput=on  SatLimitsSource=internal  UpperSaturationLimit=100  LowerSaturationLimit=-100  LinearizeAsGain=off  AntiWindupMode=clamping  Kb=1  LimitIntegrator=on  UpperIntegratorSaturationLimit=50  LowerIntegratorSaturationLimit=-50  POutMin=[]  POutMax=[]  IOutMin=[]  IOutMax=[]  DOutMin=[]  DOutMax=[]  NOutMin=[]  NOutMax=[]  SumOutMin=[]  SumOutMax=[]  SaturationOutMin=[]  SaturationOutMax=[]  PParamMin=[]  PParamMax=[]  IParamMin=[]  IParamMax=[]  DParamMin=[]  DParamMax=[]  NParamMin=[]  NParamMax=[]  KbParamMin=[]  KbParamMax=[]  KtParamMin=[]  KtParamMax=[]  KbOutMin=[]  KbOutMax=[]  KtOutMin=[]  KtOutMax=[]  IntegratorOutMin=[]  IntegratorOutMax=[]  FilterOutMin=[]  FilterOutMax=[]  SumI1OutMin=[]  SumI1OutMax=[]  SumI2OutMin=[]  SumI2OutMax=[]  SumI3OutMin=[]  SumI3OutMax=[]  SumI4OutMin=[]  SumI4OutMax=[]  SumDOutMin=[]  SumDOutMax=[]  DifferentiatorOutMin=[]  DifferentiatorOutMax=[]  FilterDiffOutCoefMin=[]  FilterDiffOutCoefMax=[]  ReciprocalOutMin=[]  ReciprocalOutMax=[]  SumDenOutMin=[]  SumDenOutMax=[]  SumNumOutMin=[]  SumNumOutMax=[]  DivideOutMin=[]  DivideOutMax=[]  UdiffTsProdOutMin=[]  UdiffTsProdOutMax=[]  NTsProdOutMin=[]  NTsProdOutMax=[]  UintegralTsProdOutMin=[]  UintegralTsProdOutMax=[]  UngainTsProdOutMin=[]  UngainTsProdOutMax=[]  ClampingZeroOutDataTypeStr=Inherit: Inherit via back propagation  ClampingZeroOutMin=[]  ClampingZeroOutMax=[]  FilterDenConstantOutDataTypeStr=Inherit: Inherit via back propagation  FilterDenConstantOutMin=[]  FilterDenConstantOutMax=[]  PCopyOutDataTypeStr=Inherit: Inherit via back propagation  PCopyOutMin=[]  PCopyOutMax=[]  NCopyOutDataTypeStr=Inherit: Inherit via back propagation  NCopyOutMin=[]  NCopyOutMax=[]  IntegratorContinuousStateAttributes=''  IntegratorStateMustResolveToSignalObject=off  IntegratorRTWStateStorageClass=Auto  FilterContinuousStateAttributes=''  FilterStateMustResolveToSignalObject=off  FilterRTWStateStorageClass=Auto  ParallelPVariant=InternalParameters  IdealPVariant=Disabled  IVariant=InternalParameters  DVariant=InternalParameters  IntegratorVariant=Discrete  SatVariant=Enabled  AWVariant=DiscClampingParallel  PCopyVariant=Disabled  TRVariant=Disabled  FdbkBlocksVariant=Forward  IdealPFdbkVariant=Disabled  SatFdbkVariant=Disabled  DerivativeFilterVariant=ForwardEulerFilter  NVariant=InternalParameters  NCopyVariant=Disabled  FilterICVariant=InternalICsFilter  IntegratorICVariant=InternalICs  ExternalResetVariant=Disabled  TRSumVariant=Passthrough  SumFdbkVariant=Disabled  SumVariant=Sum_PID  TsampFilterVariant=InternalTs  TsampNgainVariant=Passthrough  TsampIntegralVariant=Disabled_SignalSpec  ExternalSaturationOutDataTypeStr=Inherit: Same as second input  DerivativeSourceVariant=ErrorSignal  PreIntVariant=InternalPreInt
      settings: LibrarySourceBlock=simulink/Discrete/Discrete PID Controller
  Gain : Gain  Gain=0.05
  Gain1 : Gain  Gain=0.05
  Gain2 : Gain
  Gain3 : Gain  Gain=-1
  MATLAB Function : MATLAB Function  TreatAsAtomicUnit=on
  Manual Switch : ManualSwitch  Commented=on  CurrentSetting=0
  Manual Switch1 : ManualSwitch  Commented=on  CurrentSetting=0
  Python Code : PythonCode  OutputCode=|
      | import numpy as np
      | from numpy import sign
      | """
      | Reference handler for velocity controller.
      | 
      | Input: desired velocity in y-direction
      | Output: y-level reference 
      | 
      | y_ref: persistent
      | flag: persistent
      | 
      | """
      | 
      | # stick tolerance depending on expected noise level of joystick
      | stick_tolerance = 0.01
      | 
      | # desired reference change in m/s when stick is fully deflected
      | meterspersec = np.abs(stick_signal)
      | Ts = 0.01
      | 
      | ############################################################################
      | # Reference handler code
      | ############################################################################
      | 
      | import numpy as np
      | from numpy import sign
      | 
      | if flag is None:
      |     flag = 1
      | 
      | if y_ref is None:
      |     y_ref = 0
      |     
      |     
      | if mode == 1:
      |     y_ref = y_meas
      | 
      | if stick_signal < stick_tolerance and stick_signal > -stick_tolerance:
      |     stick_signal = 0
      | 
      | if stick_signal == 0 and flag == 0:
      |     y_ref = y_meas
      |     flag = 1
      | 
      | if stick_signal != 0:
      |         flag = 0
      |         y_ref += sign(stick_signal) * meterspersec * Ts 
      | 
      | y_ref_out = y_ref
  Step1 : Step  SampleTime=0.01
  Step2 : Step  Time=5  SampleTime=0.01
  Subsystem : Subsystem
  Subsystem1 : Subsystem
  Sum1 : Sum  Inputs=|+-
  Sum2 : Sum  Inputs=++|
  Sum3 : Sum  Inputs=|+-
  Sum4 : Sum  Inputs=|++
  Sum6 : Sum  Inputs=-+|
  Switch : Switch  Criteria=u2 > Threshold  SaturateOnIntegerOverflow=off  InputSameDT=off
  Switch1 : Switch  Criteria=u2 > Threshold  SaturateOnIntegerOverflow=off  InputSameDT=off
  Switch2 : Switch  Criteria=u2 > Threshold  Threshold=0.2  SaturateOnIntegerOverflow=off  InputSameDT=off
  Switch3 : Switch  Criteria=u2 > Threshold  Threshold=0.2  SaturateOnIntegerOverflow=off  InputSameDT=off
  Switch4 : Switch  Criteria=u2 > Threshold  Threshold=0.2  SaturateOnIntegerOverflow=off  InputSameDT=off
  u1 : Outport
  u2 : Outport  Port=2
  theta2dot : Outport  Port=3
  theta1dot : Outport  Port=4
  wires:
  Sum6/1 -> Discrete PID Controller4/1, Discrete PID Controller/1  "error1"
  MATLAB Function/1(thetadot_ref) -> Demux/1  "thetadot_ref"
  xdotInput/1 -> Gain/1  "xdotInput"
  ydotInput/1 -> Gain1/1  "ydotInput"
  theta1/1 -> Degrees to Radians/1  "theta1"
  theta2/1 -> Degrees to Radians1/1  "theta2"
  In1/1 -> Subsystem1/1(In2)
  Sum1/1 -> Discrete PID Controller3/1, Discrete PID Controller2/1  "error2"
  Gain/1 -> MATLAB Function/1(vx_ref)  "vx_ref"
  Gain1/1 -> Python Code/1  "vy_ref"
  In2/1 -> Subsystem/1(In2)
  Subsystem/1(thetadot2_meas) -> Sum1/2, theta2dot/1  "thetadot2_meas"
  Subsystem1/1(thetadot1_meas) -> Sum6/1, theta1dot/1  "thetadot1_meas"
  Degrees to Radians/1 -> MATLAB Function/3(theta1)
  Degrees to Radians1/1 -> MATLAB Function/4(theta2)
  Discrete PID Controller2/1 -> Switch/1
  Gain3/1 -> Sum2/2
  Discrete PID Controller/1 -> Switch1/3
  1-D Lookup Table Boom/1 -> Gain2/1
  Sum4/1 -> u2/1
  1-D Lookup Table Stick/1 -> Sum4/2
  Sum2/1 -> u1/1
  Python Code/1 -> Sum3/1  "y_ref"
  In3/1 -> Sum3/2, Python Code/2  "y_meas"
  Sum3/1 -> Switch3/3  "y_error"
  Demux/1 -> Sum6/2, 1-D Lookup Table Boom/1, Switch1/2  "theta1dot_ref"
  Demux/2 -> Switch/2, 1-D Lookup Table Stick/1, Sum1/1  "theta2dot_ref"
  Switch/1 -> Sum4/1
  Discrete PID Controller3/1 -> Switch/3
  Constant2/1 -> Manual Switch/2
  Constant3/1 -> Manual Switch1/2
  Constant/1 -> Manual Switch/1
  Constant1/1 -> Manual Switch1/1
  Discrete PID Controller4/1 -> Switch1/1
  Switch1/1 -> Gain3/1
  Gain2/1 -> Sum2/1
  Constant4/1 -> Switch3/1
  Switch3/1 -> Switch4/1  "y_error_test"
  Mode_Flag/1 -> Switch3/2, Python Code/3
  Constant5/1 -> Switch2/3
  Step1/1 -> Switch2/2
  Discrete PID Controller1/1 -> Switch2/1
  Switch2/1 -> MATLAB Function/2(vy_ref)  "vyref"
  Switch4/1 -> Discrete PID Controller1/1  "vyref"
  Step2/1 -> Switch4/2
  Constant6/1 -> Switch4/3

== system New_com_Fixed_Angle/Read Sensors/Function-Call Subsystem ==
  In1 : Inport
  function : TriggerPort  TriggerType=function-call  VariantControl=(inherit)
  CAN Unpack : canmsglib/CAN Unpack  CANdbFile=C:\Users\Viktor Traktor\Downloads\VolvoExcavator\systemIdentificationVolvo\ec20_kth.dbc  MsgList=Rot_01  MsgName=Rot_01  MsgIDType=Extended (29-bit identifier)  MsgIdentifier=419408385  MsgLength=8  SignalInfo={'SnsrPos_01','0','32','LE','unsigned','Standard','0','1','0','0','4294967295';'SnsrRPM_01','32','16','LE','unsigned','Standard','0','1','0','0','65535'}  IDPort=off  TimestampPort=off  ErrorPort=off  RemotePort=off  LengthPort=off  StatusPort=off  ApplyMinMax=off
      settings: LibrarySourceBlock=canlib/CAN Unpack  DataFormat=CANdb specified signals
  Terminator : Terminator
  Pos_01 : Outport
  wires:
  In1/1 -> CAN Unpack/1
  CAN Unpack/1 -> Pos_01/1
  CAN Unpack/2 -> Terminator/1

== system New_com_Fixed_Angle/Read Sensors/Function-Call Subsystem1 ==
  In1 : Inport
  function : TriggerPort  TriggerType=function-call  VariantControl=(inherit)
  CAN Unpack : canmsglib/CAN Unpack  CANdbFile=C:\Users\Viktor Traktor\Downloads\VolvoExcavator\systemIdentificationVolvo\ec20_kth.dbc  MsgList=Rot_20  MsgName=Rot_20  MsgIDType=Extended (29-bit identifier)  MsgIdentifier=419408416  MsgLength=8  SignalInfo={'SnsrPos_20','0','32','LE','unsigned','Standard','0','1','0','0','4294967295';'SnsrRPM_20','32','16','LE','unsigned','Standard','0','1','0','0','65535'}  IDPort=off  TimestampPort=off  ErrorPort=off  RemotePort=off  LengthPort=off  StatusPort=off  ApplyMinMax=off
      settings: LibrarySourceBlock=canlib/CAN Unpack  DataFormat=CANdb specified signals
  Terminator : Terminator
  Pos_20 : Outport
  wires:
  CAN Unpack/1 -> Pos_20/1
  In1/1 -> CAN Unpack/1
  CAN Unpack/2 -> Terminator/1

== system New_com_Fixed_Angle/Read Sensors/Function-Call Subsystem2 ==
  In1 : Inport
  function : TriggerPort  TriggerType=function-call  VariantControl=(inherit)
  CAN Unpack : canmsglib/CAN Unpack  CANdbFile=C:\Users\Viktor Traktor\Downloads\VolvoExcavator\systemIdentificationVolvo\ec20_kth.dbc  MsgList=Rot_33  MsgName=Rot_33  MsgIDType=Extended (29-bit identifier)  MsgIdentifier=419408435  MsgLength=8  SignalInfo={'SnsrPos_33','0','32','LE','unsigned','Standard','0','1','0','0','4294967295';'SnsrRPM_33','32','16','LE','unsigned','Standard','0','1','0','0','65535'}  IDPort=off  TimestampPort=off  ErrorPort=off  RemotePort=off  LengthPort=off  StatusPort=off  ApplyMinMax=off
      settings: LibrarySourceBlock=canlib/CAN Unpack  DataFormat=CANdb specified signals
  Terminator : Terminator
  Pos_33 : Outport
  wires:
  In1/1 -> CAN Unpack/1
  CAN Unpack/1 -> Pos_33/1
  CAN Unpack/2 -> Terminator/1
